simulink model "sensorsTest"  (R2019a)
settings: Solver=FixedStepAuto  StartTime=0.0  StopTime=inf  RelTol=1e-3  EnableMultiTasking=on
settings Model: SimulationMode=external  Creator=florian  LastModifiedBy=florian
settings SolverCC: PositivePriorityOrder=on
settings OptimizationCC: EnhancedBackFolding=on  PassReuseOutputArgsAs=Individual arguments  MaxStackSize=64  OptimizeBlockOrder=speed  DifferentSizesBufferReuse=on  OptimizationCustomize=off
settings DebuggingCC: ParameterTunabilityLossMsg=error
settings HardwareCC: ProdBitPerPointer=32  ProdBitPerSizeT=32  ProdBitPerPtrDiffT=32  ProdLargestAtomicInteger=Long  ProdLargestAtomicFloat=Double  ProdWordSize=32  ProdLongLongMode=on  ProdHWDeviceType=ARM Compatible->ARM Cortex
settings SFSimCC: MATLABDynamicMemAlloc=off
settings RTWCC: SystemTargetFile=ert.tlc  HardwareBoard=Raspberry Pi  TLCOptions="-aInlineSetEventsForThisBaseRateFcn=TLC_FALSE -aSuppressMultiTaskScheduler=TLC_FALSE  -aRateBasedStepFcn=0"  TemplateMakefile=ert_default_tmf  GenerateReport=on  Toolchain=GNU GCC Raspberry Pi  IncludeHyperlinkInReport=on  LaunchReport=on  GenerateTraceInfo=on  GenerateTraceReport=on  GenerateTraceReportSl=on  GenerateTraceReportSf=on  GenerateTraceReportEml=on
settings CodeAppCC: ForceParamTrailComments=on  IgnoreCustomStorageClasses=off  OperatorAnnotations=on  SimulinkDataObjDesc=on  SFDataObjDesc=on  InsertBlockDesc=on
settings ERTTargetCC: SupportContinuousTime=on  SupportVariableSizeSignals=on

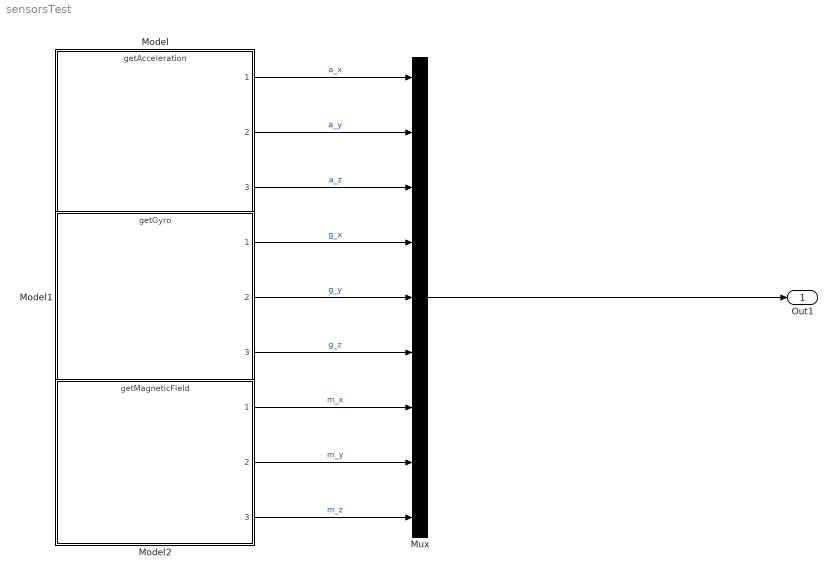
== system sensorsTest ==
  Model : ModelReference  ModelNameDialog=getAcceleration.slx  SimulationMode=Normal  ModelReferenceVersion=1.16
  Model1 : ModelReference  ModelNameDialog=getGyro.slx  SimulationMode=Normal  ModelReferenceVersion=1.6
  Model2 : ModelReference  ModelNameDialog=getMagneticField.slx  SimulationMode=Normal  ModelReferenceVersion=1.17
  Mux : Mux  Inputs=9
  Out1 : Outport
  wires:
  Model/2 -> Mux/2  "a_y"
  Model/1 -> Mux/1  "a_x"
  Model/3 -> Mux/3  "a_z"
  Model2/1 -> Mux/7  "m_x"
  Model2/2 -> Mux/8  "m_y"
  Model2/3 -> Mux/9  "m_z"
  Model1/1 -> Mux/4  "g_x"
  Model1/2 -> Mux/5  "g_y"
  Model1/3 -> Mux/6  "g_z"
  Mux/1 -> Out1/1
